simulink library "commsrccod2"  (Simulink 6.0)
settings: Solver=ode45  SolverMode=SingleTasking  StartTime=0.0  StopTime=10.0  RelTol=1e-3
libraries: dspsigattribs x8, commblksprivate x4, simulink x4, dspquant2 x2
settings Model: RequirementInfo=9  Creator=mikem  LastModifiedBy=mlongfri  ExtModeAutoUpdateStatusClock=off  ProdHWDeviceType=Specified
settings Model: ForwardingTableString=|
  | ||__slOldName__||commsrccod2/DPCM
  | Decoder||__slNewName__||cbobsv2p5/DPCM
  | Decoder||__slOldName__||commsrccod2/DPCM
  | Encoder||__slNewName__||cbobsv2p5/DPCM
  | Encoder||__slOldName__||commsrccod2/Enabled
  | Quantizer Encode||__slNewName__||cbobsv2p5/Enabled
  | Quantizer Encode||__slOldName__||commsrccod2/Quantizer
  | Decode||__slNewName__||cbobsv2p5/Quantizer
  | Decode||__slOldName__||commsrccod2/Sampled
  | Quantizer Encode||__slNewName__||cbobsv2p5/Sampled
  | Quantizer Encode
settings DataIOCC: SignalLoggingName=logsOut
settings OptimizationCC: BooleanDataType=off
settings DebuggingCC: CheckExecutionContextPreStartOutputMsg=on  CheckExecutionContextRuntimeOutputMsg=on  SolverPrmCheckMsg=none
settings HardwareCC: ProdHWDeviceType=Specified  TargetUnknown=on
settings SFSimCC: SFSimApplyToAllLibs=on  SFSimBuildMode=Incremental

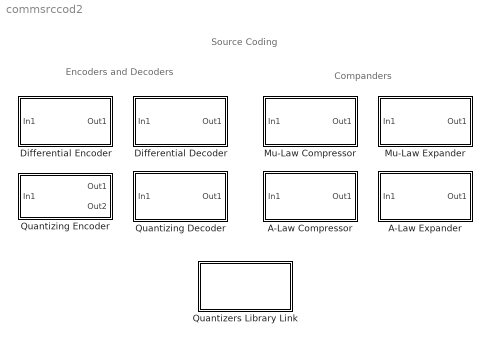
== system commsrccod2 ==
  note: Companders
  note: Encoders and Decoders
  note: Source Coding
  A-Law Compressor : Subsystem  PropExecContextAcrossSSBoundary=on  mask(A-Law Compressor){A=87.6, V=1}
      mask prompts: A "A value:"; V "Peak signal magnitude:"
      mask help:
      | Compress the input signal using A-law compression.
      |
      | The input can have any shape or frame status. This block processes each vector element independently.
      mask init:
      | lnA1=log(A)+1;AdlnA1=A/lnA1;VdlnA1=V/lnA1;VdA=V/A;AdV=A/V;
      mask Help: helpview(commbhelp)
      mask Display: disp('A-Law\nCompressor')
  A-Law Expander : Subsystem  PropExecContextAcrossSSBoundary=on  mask(A-Law Expander){A=87.6, V=1}
      mask prompts: A "A value:"; V "Peak signal magnitude:"
      mask help:
      | Expand the signal using inverse A-law compression.
      |
      | The input can have any shape or frame status. This block processes each vector element independently.
      mask init:
      | lnA1=log(A)+1;VdlnA1=V/lnA1;lnA1dA=lnA1/A;lnA1dV=lnA1/V;VdA=V/A;
      mask Help: helpview(commbhelp)
      mask Display: disp('A-Law\nExpander')
  Differential Decoder : Subsystem  PropExecContextAcrossSSBoundary=on  mask(Differential Decoder){InitCond=0}
      mask prompts: InitCond "Initial condition:"
      mask help:
      | Differentially decode the input data.
      |
      | The output of this block is the logical difference between the present input to this block and the previous input of this block.
      |
      | The input can be either a scalar or a vector.
      mask Help: helpview(commbhelp)
      mask Display: disp('Differential\nDecoder')
  Differential Encoder : Subsystem  PropExecContextAcrossSSBoundary=on  mask(Differential Encoder){InitCond=0}
      mask prompts: InitCond "Initial condition:"
      mask help:
      | Differentially encode the input data.
      |
      | The output of this block is the logical difference between the present input to this block and the previous output of this block.
      |
      | The input can be either a scalar or a vector.
      mask Help: helpview(commbhelp)
      mask Display: disp('Differential\nEncoder')
  Mu-Law Compressor : Subsystem  PropExecContextAcrossSSBoundary=on  mask(Mu-Law Compressor){mu=255, V=1}
      mask prompts: mu "mu value:"; V "Peak signal magnitude:"
      mask help:
      | Compress the input signal using mu-law compression.
      |
      | The input can have any shape or frame status. This block processes each vector element independently.
      mask init:
      | mudV=mu/V;Vln1mu=V/log(1+mu);
      mask Help: helpview(commbhelp)
      mask Display: disp('Mu-Law\nCompressor')
  Mu-Law Expander : Subsystem  PropExecContextAcrossSSBoundary=on  mask(Mu-Law Expander){mu=255, V=1}
      mask prompts: mu "mu value:"; V "Peak signal magnitude:"
      mask help:
      | Expand the signal using inverse mu-law compression.
      |
      | The input can have any shape or frame status. This block processes each vector element independently.
      mask init:
      | Vmu=V/mu;ln1mdV=log(1+mu)/V;
      mask Help: helpview(commbhelp)
      mask Display: disp('Mu-Law\nExpander')
  Quantizers Library Link : Subsystem  PropExecContextAcrossSSBoundary=on  mask{myQuantParam=0}
      mask prompts: myQuantParam "option:"
      settings: OpenFcn=commblkmorequant('dspquant');
      mask Display: disp('Quantizers\nLibrary Link');
  Quantizing Decoder : Subsystem  PropExecContextAcrossSSBoundary=on  mask(Quantizing Decoder){codebook=[-.825 -.5 0, .5 .825]}
      mask prompts: codebook "Quantization codebook:"
      mask help:
      | Decode the quantizer encoded index using a codebook.
      |
      | The input signal is the index from the Quantization codebook vector.  The input signal to be quantized can be either a scalar or a vector.
      |
      | The output signal is the quantized signal.  The values for the quantized signal are taken from the Quantization codebook vector.
      mask Help: helpview(commbhelp)
      mask Display:
      | disp('Quantizing\nDecoder')
      | port_label('input',1, 'Idx');
      | port_label('output',1,'Q(U)');
  Quantizing Encoder : Subsystem  PropExecContextAcrossSSBoundary=on  mask(Quantizing Encoder){partition=[-.75 -.25 .25 .75], codebook=[-.825 -.5 0 .5 .825]}
      mask prompts: partition "Quantization partition:"; codebook "Quantization codebook:"
      mask help:
      | Quantize the input signal using a partition and a codebook.
      |
      | The input signal is quantized according to the Quantization partition vector and encoded according to the Quantization codebook vector.  The input signal to be quantized can be either a scalar or a vector.
      |
      | The first output is the index from the Quantization codebook vector. The second output is the quantized signal.  The values for the quantized signal are taken from the Quantization codebook vector.
      mask init:
      | wsv=get_param(gcb,'MaskWSVariables');
      | partition = wsv(1).Value;
      | codebook =  wsv(2).Value;
      | 
      | partSize = size(partition);
      | CodeBkSize = size(codebook);
      | if((partSize(1) ~= 1) && (CodeBkSize(1) ~= 1))
      | 	error('The partition and the codebook must be row vectors.');
      | end
      | 
      | if(partSize(2) ~= CodeBkSize(2)-1)
      | 	error('The length of the partition vector must be one less than the length of the codebook vector.');
      | end
      mask Help: helpview(commbhelp)
      mask Display:
      | disp('Quantizing\nEncoder')
      | port_label('input',1, 'U');
      | port_label('output',1, 'Idx');
      | port_label('output',2,'Q(U)');

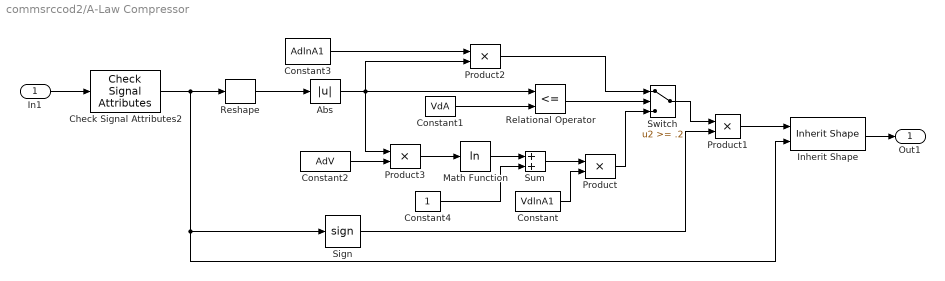
== system commsrccod2/A-Law Compressor ==
  In1 : Inport  LatchInput=off
  Abs : Abs  SaturateOnIntegerOverflow=on
  Check Signal Attributes2 : dspsigattribs/Check Signal Attributes  SigAttribCheckMethod=Matches attributes exactly  Complexity=Ignore  Frame=Ignore  DimsCheckMethod=Is...  Dimensions=Full matrix (2-D)  DatatypeCheckMethod=Ignore  DatatypeGeneral=Boolean  DtypeFloatSpecific=Any floating-point  DtypeFixedSpecific=Any fixed-point  DtypeIntSpecific=Any integer  SampleMode=Ignore
  Constant : Constant  Value=VdlnA1
  Constant1 : Constant  Value=VdA
  Constant2 : Constant  Value=AdV
  Constant3 : Constant  Value=AdlnA1
  Constant4 : Constant
  Inherit Shape : commblksprivate/Inherit Shape
  Math Function : Math  Operator=log  SaturateOnIntegerOverflow=on
  Product{,1..3} (4 alike) : Product  SaturateOnIntegerOverflow=on  InputSameDT=on
  Relational Operator : RelationalOperator  Operator=<=  LogicOutDataTypeMode=Specify via dialog  LogicDataType=float('double')  InputSameDT=on
  Reshape : simulink/Math Operations/Reshape  OutputDimensionality=1-D array  OutputDimensions=[1,1]
  Sign : Signum
  Sum : Sum  SaturateOnIntegerOverflow=on  InputSameDT=on
  Switch : Switch  Threshold=.2  SaturateOnIntegerOverflow=on  InputSameDT=on
  Out1 : Outport  InitialOutput=0
  wires:
  In1/1 -> Check Signal Attributes2/1
  Sign/1 -> Product1/2
  Switch/1 -> Product1/1
  Constant1/1 -> Relational Operator/2
  Relational Operator/1 -> Switch/2
  Product2/1 -> Switch/1
  Constant3/1 -> Product2/1
  Constant2/1 -> Product3/2
  Abs/1 -> Product3/1, Product2/2, Relational Operator/1
  Product3/1 -> Math Function/1
  Math Function/1 -> Sum/1
  Constant4/1 -> Sum/2
  Constant/1 -> Product/2
  Sum/1 -> Product/1
  Product/1 -> Switch/3
  Check Signal Attributes2/1 -> Sign/1, Inherit Shape/2, Reshape/1
  Product1/1 -> Inherit Shape/1
  Inherit Shape/1 -> Out1/1
  Reshape/1 -> Abs/1

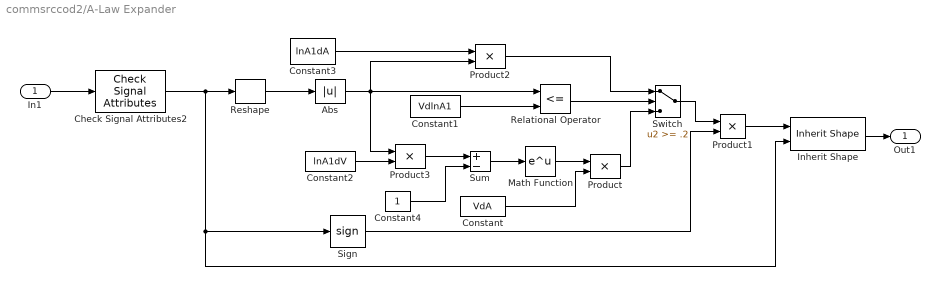
== system commsrccod2/A-Law Expander ==
  In1 : Inport  LatchInput=off
  Abs : Abs  SaturateOnIntegerOverflow=on
  Check Signal Attributes2 : dspsigattribs/Check Signal Attributes  SigAttribCheckMethod=Matches attributes exactly  Complexity=Ignore  Frame=Ignore  DimsCheckMethod=Is...  Dimensions=Full matrix (2-D)  DatatypeCheckMethod=Ignore  DatatypeGeneral=Boolean  DtypeFloatSpecific=Any floating-point  DtypeFixedSpecific=Any fixed-point  DtypeIntSpecific=Any integer  SampleMode=Ignore
  Constant : Constant  Value=VdA
  Constant1 : Constant  Value=VdlnA1
  Constant2 : Constant  Value=lnA1dV
  Constant3 : Constant  Value=lnA1dA
  Constant4 : Constant
  Inherit Shape : commblksprivate/Inherit Shape
  Math Function : Math  SaturateOnIntegerOverflow=on
  Product{,1..3} (4 alike) : Product  SaturateOnIntegerOverflow=on  InputSameDT=on
  Relational Operator : RelationalOperator  Operator=<=  LogicOutDataTypeMode=Specify via dialog  LogicDataType=float('double')  InputSameDT=on
  Reshape : simulink/Math Operations/Reshape  OutputDimensionality=1-D array  OutputDimensions=[1,1]
  Sign : Signum
  Sum : Sum  Inputs=+-  SaturateOnIntegerOverflow=on  InputSameDT=on
  Switch : Switch  Threshold=.2  SaturateOnIntegerOverflow=on  InputSameDT=on
  Out1 : Outport  InitialOutput=0
  wires:
  Product/1 -> Switch/3
  Constant/1 -> Product/2
  Constant4/1 -> Sum/2
  Constant2/1 -> Product3/2
  Constant3/1 -> Product2/1
  Product2/1 -> Switch/1
  Abs/1 -> Product3/1, Product2/2, Relational Operator/1
  Relational Operator/1 -> Switch/2
  Constant1/1 -> Relational Operator/2
  Switch/1 -> Product1/1
  Sign/1 -> Product1/2
  In1/1 -> Check Signal Attributes2/1
  Product3/1 -> Sum/1
  Sum/1 -> Math Function/1
  Math Function/1 -> Product/1
  Check Signal Attributes2/1 -> Sign/1, Inherit Shape/2, Reshape/1
  Product1/1 -> Inherit Shape/1
  Inherit Shape/1 -> Out1/1
  Reshape/1 -> Abs/1

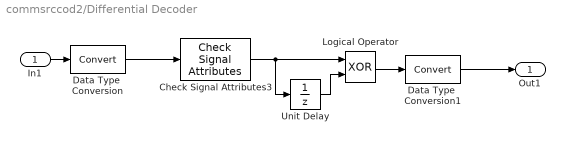
== system commsrccod2/Differential Decoder ==
  In1 : Inport  LatchInput=off
  Check Signal Attributes3 : dspsigattribs/Check Signal Attributes  SigAttribCheckMethod=Matches attributes exactly  Complexity=Ignore  Frame=Ignore  DimsCheckMethod=Is...  Dimensions=Full matrix (2-D)  DatatypeCheckMethod=Ignore  DatatypeGeneral=Boolean  DtypeFloatSpecific=Any floating-point  DtypeFixedSpecific=Any fixed-point  DtypeIntSpecific=Any integer  SampleMode=Ignore
  Data Type  Conversion : DataTypeConversion  OutDataTypeMode=boolean  SaturateOnIntegerOverflow=on  RndMeth=Zero
  Data Type  Conversion1 : DataTypeConversion  OutDataTypeMode=double  SaturateOnIntegerOverflow=on  RndMeth=Zero
  Logical Operator : Logic  Operator=XOR  LogicDataType=float('double')
  Unit Delay : UnitDelay  X0=InitCond  SampleTime=-1
  Out1 : Outport  InitialOutput=0
  wires:
  Check Signal Attributes3/1 -> Logical Operator/1, Unit Delay/1
  Unit Delay/1 -> Logical Operator/2
  In1/1 -> Data Type  Conversion/1
  Logical Operator/1 -> Data Type  Conversion1/1
  Data Type  Conversion/1 -> Check Signal Attributes3/1
  Data Type  Conversion1/1 -> Out1/1

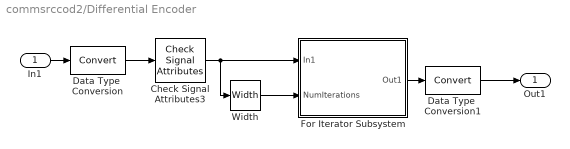
== system commsrccod2/Differential Encoder ==
  In1 : Inport  LatchInput=off
  Check Signal Attributes3 : dspsigattribs/Check Signal Attributes  SigAttribCheckMethod=Matches attributes exactly  Complexity=Ignore  Frame=Ignore  DimsCheckMethod=Is...  Dimensions=Full matrix (2-D)  DatatypeCheckMethod=Ignore  DatatypeGeneral=Boolean  DtypeFloatSpecific=Any floating-point  DtypeFixedSpecific=Any fixed-point  DtypeIntSpecific=Any integer  SampleMode=Ignore
  Data Type  Conversion : DataTypeConversion  OutDataTypeMode=boolean  SaturateOnIntegerOverflow=on  RndMeth=Zero
  Data Type  Conversion1 : DataTypeConversion  OutDataTypeMode=double  SaturateOnIntegerOverflow=on  RndMeth=Zero
  For Iterator Subsystem : Subsystem  TreatAsAtomicUnit=on  PropExecContextAcrossSSBoundary=on
  Width : Width
  Out1 : Outport
  wires:
  For Iterator Subsystem/1(Out1) -> Data Type  Conversion1/1
  In1/1 -> Data Type  Conversion/1
  Width/1 -> For Iterator Subsystem/2(NumIterations)
  Check Signal Attributes3/1 -> Width/1, For Iterator Subsystem/1(In1)
  Data Type  Conversion/1 -> Check Signal Attributes3/1
  Data Type  Conversion1/1 -> Out1/1

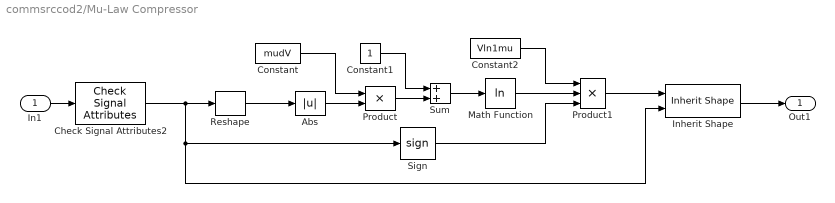
== system commsrccod2/Mu-Law Compressor ==
  In1 : Inport  LatchInput=off
  Abs : Abs  SaturateOnIntegerOverflow=on
  Check Signal Attributes2 : dspsigattribs/Check Signal Attributes  SigAttribCheckMethod=Matches attributes exactly  Complexity=Ignore  Frame=Ignore  DimsCheckMethod=Is...  Dimensions=Full matrix (2-D)  DatatypeCheckMethod=Ignore  DatatypeGeneral=Boolean  DtypeFloatSpecific=Any floating-point  DtypeFixedSpecific=Any fixed-point  DtypeIntSpecific=Any integer  SampleMode=Ignore
  Constant : Constant  Value=mudV
  Constant1 : Constant
  Constant2 : Constant  Value=Vln1mu
  Inherit Shape : commblksprivate/Inherit Shape
  Math Function : Math  Operator=log  SaturateOnIntegerOverflow=on
  Product : Product  SaturateOnIntegerOverflow=on  InputSameDT=on
  Product1 : Product  Inputs=3  SaturateOnIntegerOverflow=on  InputSameDT=on
  Reshape : simulink/Math Operations/Reshape  OutputDimensionality=1-D array  OutputDimensions=[1,1]
  Sign : Signum
  Sum : Sum  SaturateOnIntegerOverflow=on  InputSameDT=on
  Out1 : Outport  InitialOutput=0
  wires:
  Constant2/1 -> Product1/1
  Sign/1 -> Product1/3
  Math Function/1 -> Product1/2
  In1/1 -> Check Signal Attributes2/1
  Sum/1 -> Math Function/1
  Constant1/1 -> Sum/1
  Product/1 -> Sum/2
  Constant/1 -> Product/1
  Abs/1 -> Product/2
  Check Signal Attributes2/1 -> Sign/1, Inherit Shape/2, Reshape/1
  Product1/1 -> Inherit Shape/1
  Inherit Shape/1 -> Out1/1
  Reshape/1 -> Abs/1

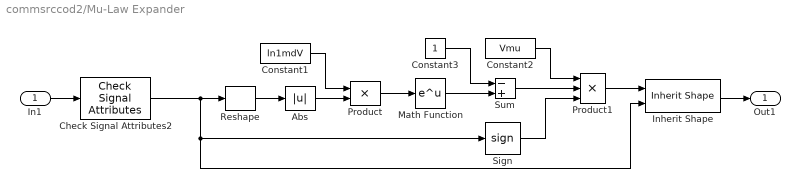
== system commsrccod2/Mu-Law Expander ==
  In1 : Inport  LatchInput=off
  Abs : Abs  SaturateOnIntegerOverflow=on
  Check Signal Attributes2 : dspsigattribs/Check Signal Attributes  SigAttribCheckMethod=Matches attributes exactly  Complexity=Ignore  Frame=Ignore  DimsCheckMethod=Is...  Dimensions=Full matrix (2-D)  DatatypeCheckMethod=Ignore  DatatypeGeneral=Boolean  DtypeFloatSpecific=Any floating-point  DtypeFixedSpecific=Any fixed-point  DtypeIntSpecific=Any integer  SampleMode=Ignore
  Constant1 : Constant  Value=ln1mdV
  Constant2 : Constant  Value=Vmu
  Constant3 : Constant
  Inherit Shape : commblksprivate/Inherit Shape
  Math Function : Math  SaturateOnIntegerOverflow=on
  Product : Product  SaturateOnIntegerOverflow=on  InputSameDT=on
  Product1 : Product  Inputs=3  SaturateOnIntegerOverflow=on  InputSameDT=on
  Reshape : simulink/Math Operations/Reshape  OutputDimensionality=1-D array  OutputDimensions=[1,1]
  Sign : Signum
  Sum : Sum  Inputs=-+  SaturateOnIntegerOverflow=on  InputSameDT=on
  Out1 : Outport  InitialOutput=0
  wires:
  Constant3/1 -> Sum/1
  Sum/1 -> Product1/2
  Math Function/1 -> Sum/2
  Sign/1 -> Product1/3
  In1/1 -> Check Signal Attributes2/1
  Constant2/1 -> Product1/1
  Product/1 -> Math Function/1
  Abs/1 -> Product/2
  Constant1/1 -> Product/1
  Check Signal Attributes2/1 -> Sign/1, Inherit Shape/2, Reshape/1
  Product1/1 -> Inherit Shape/1
  Inherit Shape/1 -> Out1/1
  Reshape/1 -> Abs/1

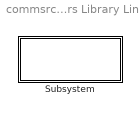
== system commsrccod2/Quantizers Library Link ==
  Subsystem : Subsystem  PropExecContextAcrossSSBoundary=on
      mask Display: disp(' ')

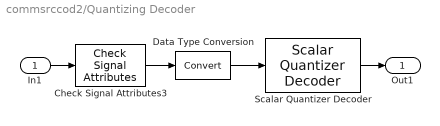
== system commsrccod2/Quantizing Decoder ==
  In1 : Inport  LatchInput=off
  Check Signal Attributes3 : dspsigattribs/Check Signal Attributes  SigAttribCheckMethod=Matches attributes exactly  Complexity=Ignore  Frame=Ignore  DimsCheckMethod=Is...  Dimensions=Full matrix (2-D)  DatatypeCheckMethod=Ignore  DatatypeGeneral=Boolean  DtypeFloatSpecific=Any floating-point  DtypeFixedSpecific=Any fixed-point  DtypeIntSpecific=Any integer  SampleMode=Ignore
  Data Type Conversion : DataTypeConversion  OutDataTypeMode=uint32  SaturateOnIntegerOverflow=on  RndMeth=Zero
  Scalar Quantizer Decoder : dspquant2/Scalar Quantizer Decoder  CBsource=Specify via dialog  invalidin=Clip  codebook=codebook  dataType=double  isSigned=on  wordLen=16  udDataType=sfix(16)  fracBitsMode=Best precision  numFracBits=11
  Out1 : Outport  InitialOutput=0
  wires:
  Scalar Quantizer Decoder/1 -> Out1/1
  In1/1 -> Check Signal Attributes3/1
  Check Signal Attributes3/1 -> Data Type Conversion/1
  Data Type Conversion/1 -> Scalar Quantizer Decoder/1

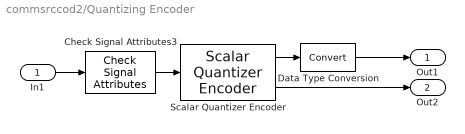
== system commsrccod2/Quantizing Encoder ==
  In1 : Inport  LatchInput=off
  Check Signal Attributes3 : dspsigattribs/Check Signal Attributes  SigAttribCheckMethod=Matches attributes exactly  Complexity=Ignore  Frame=Ignore  DimsCheckMethod=Is...  Dimensions=Full matrix (2-D)  DatatypeCheckMethod=Ignore  DatatypeGeneral=Boolean  DtypeFloatSpecific=Any floating-point  DtypeFixedSpecific=Any fixed-point  DtypeIntSpecific=Any integer  SampleMode=Ignore
  Data Type Conversion : DataTypeConversion  OutDataTypeMode=double  SaturateOnIntegerOverflow=on  RndMeth=Zero
  Scalar Quantizer Encoder : dspquant2/Scalar Quantizer Encoder  paramSrc=Specify via dialog  partType=Unbounded  BBoundary=[1:10]  UBoundary=partition  SearchMethod=Linear  tieBreakRule=Choose the lower index  outQU=on  outQError=off  codebook=codebook  outStatus=off  invalidin=Clip  idtype=int32  roundingMode=Floor  overflowMode=off
  Out1 : Outport  InitialOutput=0
  Out2 : Outport  Port=2  InitialOutput=0
  wires:
  Scalar Quantizer Encoder/2 -> Out2/1
  Scalar Quantizer Encoder/1 -> Data Type Conversion/1
  In1/1 -> Check Signal Attributes3/1
  Check Signal Attributes3/1 -> Scalar Quantizer Encoder/1
  Data Type Conversion/1 -> Out1/1

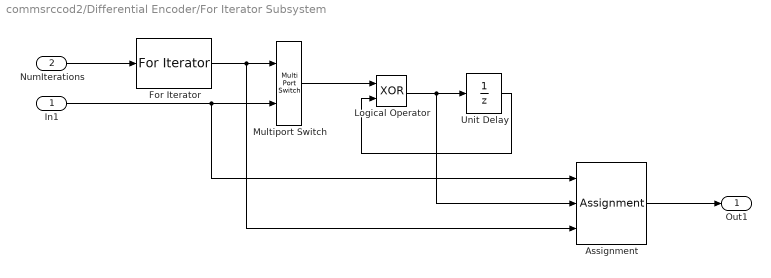
== system commsrccod2/Differential Encoder/For Iterator Subsystem ==
  In1 : Inport  LatchInput=off
  NumIterations : Inport  Port=2  LatchInput=off
  Assignment : Assignment  ElementSrc=External
  For Iterator : ForIterator  IterationSource=external
  Logical Operator : Logic  Operator=XOR  AllPortsSameDT=off
  Multiport Switch : MultiPortSwitch  Inputs=1  SaturateOnIntegerOverflow=on
  Unit Delay : UnitDelay  X0=InitCond  SampleTime=-1
  Out1 : Outport
  wires:
  In1/1 -> Assignment/1, Multiport Switch/2
  Assignment/1 -> Out1/1
  Unit Delay/1 -> Logical Operator/2
  Logical Operator/1 -> Assignment/2, Unit Delay/1
  Multiport Switch/1 -> Logical Operator/1
  For Iterator/1 -> Assignment/3, Multiport Switch/1
  NumIterations/1 -> For Iterator/1

== system commsrccod2/Quantizers Library Link/Subsystem ==
